simulink model "OpenLoopSys"  (R2019a)
settings: Solver=VariableStepAuto  StartTime=0.0  StopTime=25  RelTol=1e-3
settings Model: Creator=Fiona Lin  LastModifiedBy=Fiona Lin

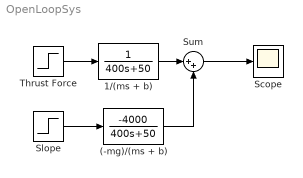
== system OpenLoopSys ==
  "(-mg)/(ms + b) " : TransferFcn  Numerator=-4000  Denominator=[400 50]
  1/(ms + b) : TransferFcn  Denominator=[400 50]
  Scope : Scope
  "Slope " : Step  Time=10  After=0.1  SampleTime=0
  Sum : Sum  Inputs=|++
  "Thrust Force " : Step  Time=2  After=500  SampleTime=0
  wires:
  1/(ms + b)/1 -> Sum/1
  "(-mg)/(ms + b) "/1 -> Sum/2
  "Thrust Force "/1 -> 1/(ms + b)/1
  "Slope "/1 -> "(-mg)/(ms + b) "/1
  Sum/1 -> Scope/1
